simulink model "sim_pizeo_T005_epison005"  (R2022b)
settings: Solver=FixedStepAuto  StartTime=0.0  StopTime=5  FixedStep=0.001  RelTol=1e-3  EnableMultiTasking=on
settings Model: Creator=Administrator  LastModifiedBy=huheyu
settings SolverCC: AlgebraicLoopSolver=TrustRegion
settings DataIOCC: LimitDataPoints=on  SaveFormat=Array  ReturnWorkspaceOutputs=off
settings OptimizationCC: LifeSpan=inf
settings DebuggingCC: UnderspecifiedInitializationDetection=Classic  MergeDetectMultiDrivingBlocksExec=none  SolverPrmCheckMsg=warning  UnconnectedInputMsg=warning  UnconnectedOutputMsg=warning  UnconnectedLineMsg=warning  StateNameClashWarn=warning  SFUnexpectedBacktrackingDiag=warning  SFNoUnconditionalDefaultTransitionDiag=warning  SFExecutionAtInitializationDiag=none  ArithmeticOperatorsInVariantConditions=warning
settings HardwareCC: ProdBitPerPointer=32  ProdBitPerSizeT=32  ProdBitPerPtrDiffT=32  ProdLargestAtomicFloat=None  ProdIntDivRoundTo=Undefined  ProdEndianess=Unspecified  ProdWordSize=32  ProdHWDeviceType=32-bit Generic
settings ModelReferenceCC: EnableRefExpFcnMdlSchedulingChecks=on  PropagateSignalLabelsOutOfModel=off
settings SFSimCC: SimUseLocalCustomCode=off  CustomCodeUndefinedFunction=UseInterfaceOnly
settings RTWCC: RTWUseLocalCustomCode=off  DLArmComputeVersion=19.05
settings CodeAppCC: StateflowObjectComments=on
settings GRTTargetCC: TargetLangStandard=C89/C90 (ANSI)
settings ConfigComp: CovMetricSettings=dw  CovSaveCumulativeToWorkspaceVar=on  CovSaveSingleToWorkspaceVar=on  CovExternalEMLEnable=off

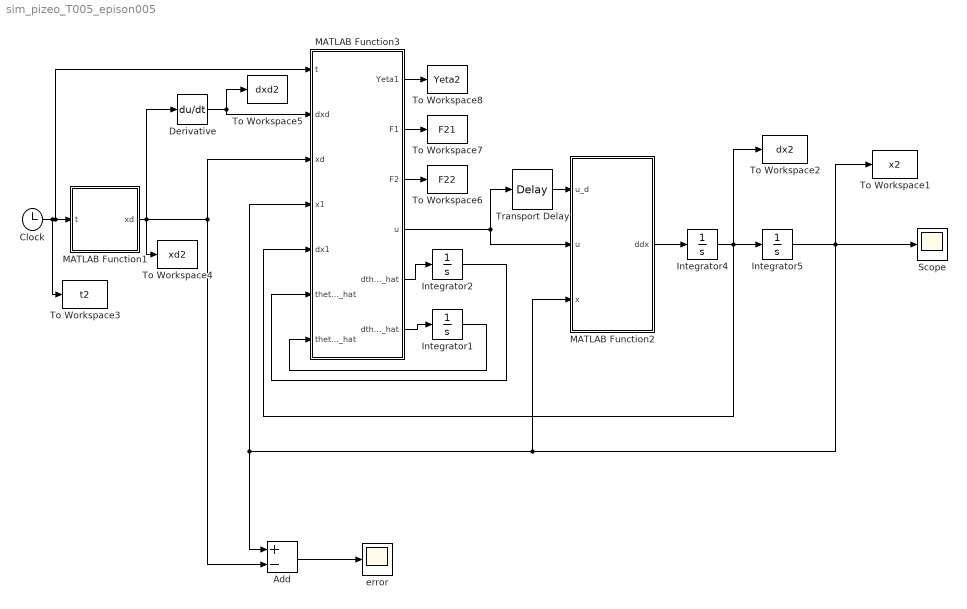
== system sim_pizeo_T005_epison005 ==
  Add : Sum  Inputs=+-
  Clock : Clock
  Derivative : Derivative
  Integrator{1..2,4..5} (4 alike) : Integrator
  MATLAB Function1 : MATLAB Function  TreatAsAtomicUnit=on
  MATLAB Function2 : MATLAB Function  TreatAsAtomicUnit=on
  MATLAB Function3 : MATLAB Function  TreatAsAtomicUnit=on
  Scope : Scope
  To Workspace1 : ToWorkspace  VariableName=x2  SampleTime=-1
  To Workspace2 : ToWorkspace  VariableName=dx2  SampleTime=-1
  To Workspace3 : ToWorkspace  VariableName=t2  SampleTime=-1
  To Workspace4 : ToWorkspace  VariableName=xd2  SampleTime=-1
  To Workspace5 : ToWorkspace  VariableName=dxd2  SampleTime=-1
  To Workspace6 : ToWorkspace  VariableName=F22  SampleTime=-1
  To Workspace7 : ToWorkspace  VariableName=F21  SampleTime=-1
  To Workspace8 : ToWorkspace  VariableName=Yeta2  SampleTime=-1
  Transport Delay : TransportDelay  DelayTime=0.001
  error : Scope
  wires:
  Clock/1 -> To Workspace3/1, MATLAB Function1/1(t), MATLAB Function3/1(t)
  MATLAB Function1/1(xd) -> Add/2, MATLAB Function3/3(xd), Derivative/1, To Workspace4/1
  Integrator5/1 -> To Workspace1/1, Scope/1, MATLAB Function2/3(x), MATLAB Function3/4(x1), Add/1
  Derivative/1 -> To Workspace5/1, MATLAB Function3/2(dxd)
  MATLAB Function2/1(ddx) -> Integrator4/1
  MATLAB Function3/4(u) -> Transport Delay/1, MATLAB Function2/2(u)
  Add/1 -> error/1
  Transport Delay/1 -> MATLAB Function2/1(u_d)
  Integrator1/1 -> MATLAB Function3/7(theta2_hat)
  MATLAB Function3/6(dtheta2_hat) -> Integrator1/1
  MATLAB Function3/5(dtheta1_hat) -> Integrator2/1
  Integrator2/1 -> MATLAB Function3/6(theta1_hat)
  Integrator4/1 -> MATLAB Function3/5(dx1), To Workspace2/1, Integrator5/1
  MATLAB Function3/3(F2) -> To Workspace6/1
  MATLAB Function3/2(F1) -> To Workspace7/1
  MATLAB Function3/1(Yeta1) -> To Workspace8/1

== matlab function sim_pizeo_T005_epison005/MATLAB Function1 ==
  data: t input; xd output
function xd= getxx(t)
xd=sin(2*pi*t);

== matlab function sim_pizeo_T005_epison005/MATLAB Function3 ==
  data: Yeta1 output; F1 output; F2 output; t input; dxd input; u output; xd input; x1 input; dx1 input; theta1_hat input; theta2_hat input; dtheta1_hat output; dtheta2_hat output
function [Yeta1,F1,F2,u,dtheta1_hat,dtheta2_hat]= getxx(t,dxd,xd,x1,dx1,theta1_hat,theta2_hat)


T=0.05; epison=0.05;
k1=30;k2=100;r1=0.5;r2=0.1;

if t<T-0.01
    Yeta1=(1/(t+0.01)-1/T)^3+epison;
    if Yeta1>10
        Yeta1=100;
    end
else
    Yeta1=epison;
end
e=x1-xd;
h11=1-(e/Yeta1)^2;


F1=3;F2=10;
h12=1-(x1/F1)^2;
h2=1-(dx1/F2)^2;
h1=h11*h12/(h11+h12);
%h1=h11;
%h2=1;

ksi1=e/h1;
ksi2=dx1/h2;
mu1=1/h1;
mu2=1/h2;

z1=ksi1;
ci1=[0 0 0 0]';
xi1=[x1,xd,dx1,dxd]';

fai1=exp(-(xi1-ci1)'*(xi1-ci1)/4);
faic1=fai1*fai1+1;


alpha1=1/h2*(-k1*z1+dxd-r1*mu1*theta1_hat*faic1*z1);
dtheta1_hat=-r1*theta1_hat+r1*mu1*mu1*faic1*z1*z1;

ci2=[0 0 0 0]';
xi2=[x1,xd,dx1,dxd]';
fai2=exp(-(xi2-ci2)'*(xi2-ci2)/4);
faic2=fai2*fai2+1;

z2=ksi2-alpha1;
dtheta2_hat=-r2*theta2_hat+r2*mu2*mu2*z2*z2*faic2;

u=-k2*z2-0*1/mu2*mu1*mu1*h2*h2*z1*z1*z2-r2*mu2*theta2_hat*faic1*z2;











%u=-100*(x-xd)-200*(dx-dxd);

== matlab function sim_pizeo_T005_epison005/MATLAB Function2 ==
  data: u_d input; u input; ddx output; x input
function ddx= getxx(u_d,u,x)



   r=0.6;
   rho=10*tanh(u);
   fr=max(rho-r,min(rho+r,u_d));
   pr=0.6*exp(-0.108*(r-0.5)^2);
   w1=0.45*u+fr*pr;
   w=double(w1);

ddx=-0.5*sin(x)+0.01*cos(5*x)+w;
